simulink model "quadrotor"  (R2016b)
settings: Solver=ode4  StartTime=0.0  StopTime=50  FixedStep=0.01  RelTol=1e-3  EnableMultiTasking=on
values from neighbouring files (symbols this model uses):
  a = 6378137    [Quadparameters.m]
  b = 6356752.3142    [Quadparameters.m]
  d = 7.5*10^(-7)    (= 7.5e-07)    [Quadparameters.m]
  g = 9.81    [Quadparameters.m]
  Ix = 7.5*10^(-3)    (= 0.0075)    [Quadparameters.m]
  Iy = 7.5*10^(-3)    (= 0.0075)    [Quadparameters.m]
  Iz = 1.3*10^(-2)    (= 0.013)    [Quadparameters.m]
  Jr = 6.5*10^(-5)    (= 6.5e-05)    [Quadparameters.m]
  kdp = 0.4    [Quadparameters.m]
  kdps = 0.4    [Quadparameters.m]
  kdt = 0.4    [Quadparameters.m]
  kdz = 20    [Quadparameters.m]
  kpp = 0.8    [Quadparameters.m]
  kpps = 1    [Quadparameters.m]
  kpt = 1.2    [Quadparameters.m]
  kpz = 100    [Quadparameters.m]
  l = 0.23    [Quadparameters.m]
  m = 0.65    [Quadparameters.m]
  NEDDownECEF = [-cos(StartLat)*cos(StartLong) -cos(StartLat)*sin(StartLong) -sin(StartLat)*cos(StartLong)]    [Quadparameters.m]
  NEDEastECEF = [-sin(StartLong) cos(StartLong) 0]    [Quadparameters.m]
  NEDNorthECEF = [-sin(StartLat) 0 cos(StartLat)]    [Quadparameters.m]
  StartECEFX = (a/(sqrt(cos(StartLat)*cos(StartLat)+(b^2/a^2)*sin(StartLat)*sin(StartLat)))+ StartAlt)*cos(StartLat)*cos(StartLong)    [Quadparameters.m]
  StartECEFY = (a/(sqrt(cos(StartLat)*cos(StartLat)+(b^2/a^2)*sin(StartLat)*sin(StartLat)))+ StartAlt)*cos(StartLat)*sin(StartLong)    [Quadparameters.m]
  StartECEFZ = (b/(sqrt((a^2/b^2)*cos(StartLat)*cos(StartLat)+sin(StartLat)*sin(StartLat)))+ StartAlt)*sin(StartLat)    [Quadparameters.m]
undefined symbols (not defined in the file or in its folder): AirSpeed, Altitude, Heading, Latitude, Longitude, Pitch, Roll, VertSpeed
settings Model: ParamWorkspaceSource=ReferencedWorkspace  TunableVars=Ep,Eps,Et,Ez,Gains,Ix,Iy,Iz,Jr,Kdp,Kdps,Kdt,Kdz,Kpp,Kpps,Kpt,Kpz,PhidF,Phiinit,PsidF,Psiinit,ThetadF,Thetainit,Ufour,Uone,Uthree,Utwo,ZdF,Zinit,b,d,g,kdp,kdps,kdt,kdz,kpp,kpps,kpt,kpz,l,m,phitime,psitime,thetatime,tout,yout,ztime  TunableVarsStorageClass=Auto,Auto,Auto,Auto,Auto,Auto,Auto,Auto,Auto,Auto,Auto,Auto,Auto,Auto,Auto,Auto,Auto,Auto,Auto,Auto,Auto,Auto,Auto,Auto,Auto,Auto,Auto,Auto,Auto,Auto,Auto,Auto,Auto,Auto,Auto,Auto,Auto,Auto,Auto,Auto,Auto,Auto,Auto,Auto,Auto,Auto,Auto,Auto  TunableVarsTypeQualifier=,,,,,,,,,,,,,,,,,,,,,,,,,,,,,,,,,,,,,,,,,,,,,,,  Creator=dura_um  LastModifiedBy=leim_ni
settings DataIOCC: LimitDataPoints=on  SaveFormat=Array  SignalLoggingSaveFormat=ModelDataLogs  SaveOutput=off  SignalLogging=off  SaveTime=off
settings OptimizationCC: DefaultParameterBehavior=Inlined  ExpressionDepthLimit=2147483647  InitFltsAndDblsToZero=on  LifeSpan=inf
settings DebuggingCC: UnderspecifiedInitializationDetection=Classic  MergeDetectMultiDrivingBlocksExec=none  SolverPrmCheckMsg=warning  FcnCallInpInsideContextMsg=warning  StateNameClashWarn=warning  StrictBusMsg=Warning  SFUnexpectedBacktrackingDiag=warning  SFNoUnconditionalDefaultTransitionDiag=warning  SFExecutionAtInitializationDiag=none
settings HardwareCC: ProdBitPerPointer=32  ProdBitPerSizeT=32  ProdBitPerPtrDiffT=32  ProdLargestAtomicFloat=None  ProdIntDivRoundTo=Undefined  ProdEndianess=Unspecified  ProdWordSize=32  ProdHWDeviceType=32-bit Generic
settings ModelReferenceCC: PropagateSignalLabelsOutOfModel=off
settings RTWCC: SystemTargetFile=grt_2Simulate.tlc  GenerateMakefile=off  TemplateMakefile=grt_2Simulate_msvc.tmf  Description=2Simulate Target  TargetLang=C++
settings STFCustomTargetCC: ModelReferenceCompliant=off  GeneratePreprocessorConditionals=Disable all  CPPClassGenCompliant=on  SystemTargetFile=grt_2Simulate.tlc
settings GRTTargetCC: TargetLangStandard=C89/C90 (ANSI)  ModelReferenceCompliant=off  ParMdlRefBuildCompliant=off  CompOptLevelCompliant=off  ConcurrentExecutionCompliant=off  GeneratePreprocessorConditionals=Disable all  CombineOutputUpdateFcns=off  MatFileLogging=off  GRTInterface=on  UseToolchainInfoCompliant=off  ExtModeMexFile=noextcomm
settings ConfigComp: CovMetricSettings=dw  CovHtmlReporting=on  CovSaveCumulativeToWorkspaceVar=on  CovSaveSingleToWorkspaceVar=on  CovExternalEMLEnable=off

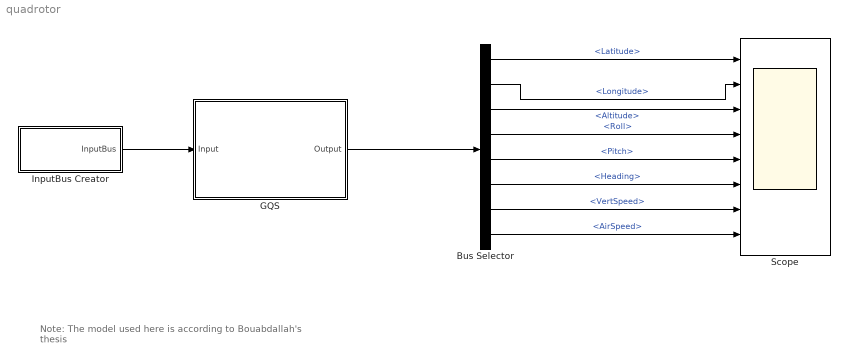
== system quadrotor ==
  note: Note:
      | The model used here is according to Bouabdallah's thesis
  Bus Selector : BusSelector  OutputSignals=Latitude,Longitude,Altitude,Roll,Pitch,Heading,VertSpeed,AirSpeed
  GQS : Subsystem
  "InputBus Creator " : Subsystem
  Scope : Scope  NumInputPorts=8
  wires:
  "InputBus Creator "/1(InputBus) -> GQS/1(Input)
  GQS/1(Output) -> Bus Selector/1
  Bus Selector/3 -> Scope/3  "<Altitude>"
  Bus Selector/4 -> Scope/4  "<Roll>"
  Bus Selector/5 -> Scope/5  "<Pitch>"
  Bus Selector/6 -> Scope/6  "<Heading>"
  Bus Selector/1 -> Scope/1  "<Latitude>"
  Bus Selector/2 -> Scope/2  "<Longitude>"
  Bus Selector/7 -> Scope/7  "<VertSpeed>"
  Bus Selector/8 -> Scope/8  "<AirSpeed>"

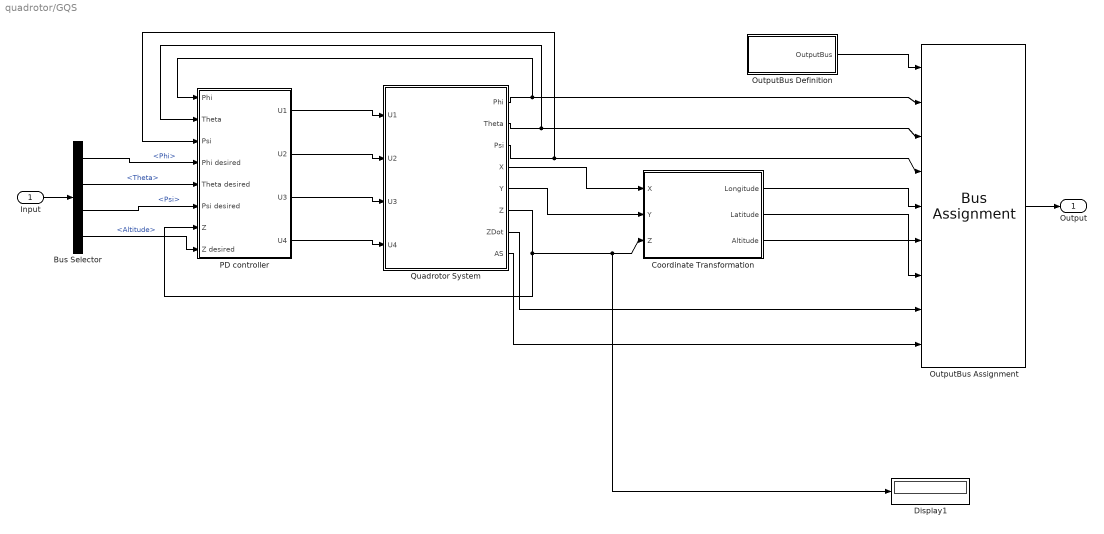
== system quadrotor/GQS ==
  Input : Inport  OutDataTypeStr=Bus: InputVector
  Bus Selector : BusSelector  OutputSignals=Phi,Theta,Psi,Altitude
  Coordinate Transformation : Subsystem
  Display1 : Display
  OutputBus Assignment : BusAssignment  AssignedSignals=Roll,Pitch,Heading,Longitude,Latitude,Altitude,VertSpeed,AirSpeed
  OutputBus Definition : Subsystem
  PD controller : Subsystem
  Quadrotor System : Subsystem
  Output : Outport  OutDataTypeStr=Bus: OutputVector
  wires:
  Quadrotor System/1(Phi) -> PD controller/1(Phi), OutputBus Assignment/2
  Quadrotor System/2(Theta) -> PD controller/2(Theta), OutputBus Assignment/3
  Quadrotor System/6(Z) -> PD controller/7(Z), Display1/1, Coordinate Transformation/3(Z)
  Quadrotor System/3(Psi) -> PD controller/3(Psi), OutputBus Assignment/4
  Bus Selector/4 -> PD controller/8(Z desired)  "<Altitude>"
  PD controller/1(U1) -> Quadrotor System/1(U1)
  OutputBus Assignment/1 -> Output/1
  Bus Selector/1 -> PD controller/4(Phi desired)  "<Phi>"
  Quadrotor System/4(X) -> Coordinate Transformation/1(X)
  OutputBus Definition/1(OutputBus) -> OutputBus Assignment/1
  Quadrotor System/5(Y) -> Coordinate Transformation/2(Y)
  Input/1 -> Bus Selector/1
  Coordinate Transformation/1(Longitude) -> OutputBus Assignment/5
  Coordinate Transformation/3(Altitude) -> OutputBus Assignment/7
  Coordinate Transformation/2(Latitude) -> OutputBus Assignment/6
  PD controller/2(U2) -> Quadrotor System/2(U2)
  PD controller/4(U4) -> Quadrotor System/4(U4)
  Bus Selector/2 -> PD controller/5(Theta desired)  "<Theta>"
  PD controller/3(U3) -> Quadrotor System/3(U3)
  Bus Selector/3 -> PD controller/6(Psi desired)  "<Psi>"
  Quadrotor System/7(ZDot) -> OutputBus Assignment/8
  Quadrotor System/8(AS) -> OutputBus Assignment/9

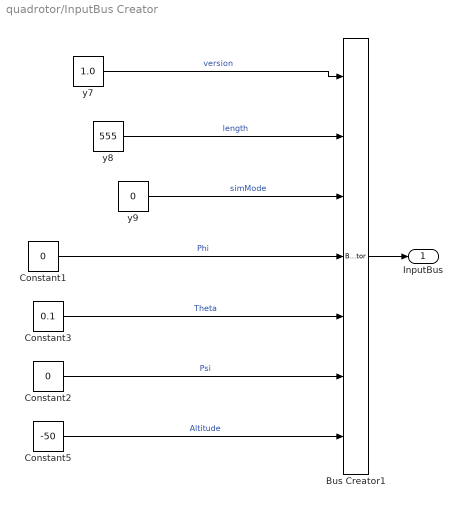
== system quadrotor/InputBus Creator  ==
  Bus Creator1 : BusCreator  Inputs='version','length','simMode','Phi','Theta','Psi','Altitude'  OutDataTypeStr=Bus: InputVector
  Constant1 : Constant  Value=0
  Constant2 : Constant  Value=0
  Constant3 : Constant  Value=0.1
  Constant5 : Constant  Value=-50
  y7 : Constant  Value=1.0  OutDataTypeStr=double
  y8 : Constant  Value=555  OutDataTypeStr=double
  y9 : Constant  Value=0  OutDataTypeStr=double
  InputBus : Outport  OutDataTypeStr=Bus: InputVector
  wires:
  Constant1/1 -> Bus Creator1/4  "Phi"
  Constant3/1 -> Bus Creator1/5  "Theta"
  Constant2/1 -> Bus Creator1/6  "Psi"
  Constant5/1 -> Bus Creator1/7  "Altitude"
  Bus Creator1/1 -> InputBus/1
  y9/1 -> Bus Creator1/3  "simMode"
  y8/1 -> Bus Creator1/2  "length"
  y7/1 -> Bus Creator1/1  "version"

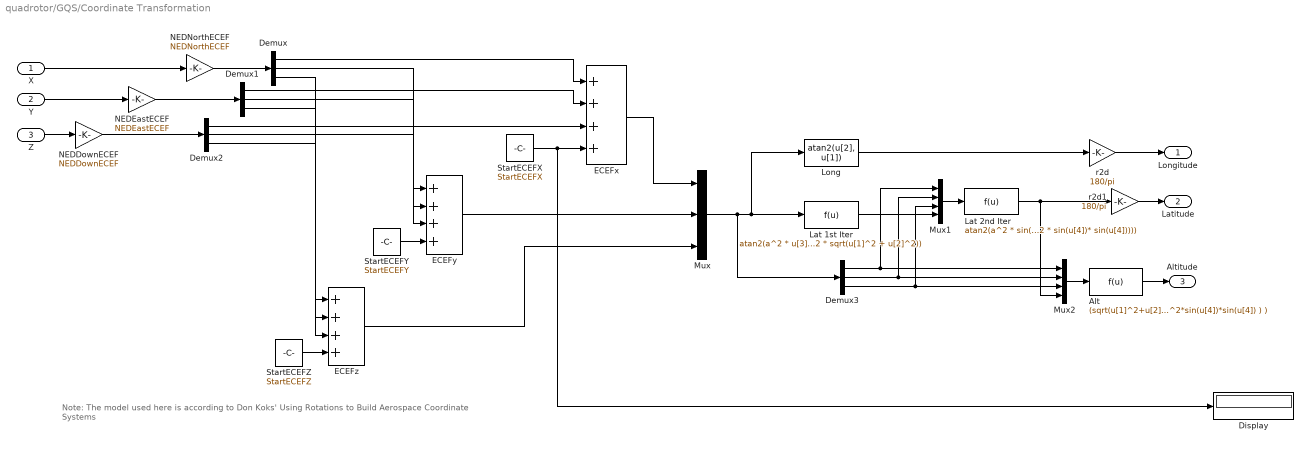
== system quadrotor/GQS/Coordinate Transformation ==
  note: Note:
      | The model used here is according to Don Koks' Using Rotations to Build Aerospace Coordinate Systems
  X : Inport
  Y : Inport  Port=2
  Z : Inport  Port=3
  Alt : Fcn  Expr=(sqrt(u[1]^2+u[2]^2)/cos(u[4]))-( a^2 / sqrt( a^2 * cos(u[4])*cos(u[4])+b^2*sin(u[4])*sin(u[4]) ) )
  Demux{,1..3} (4 alike) : Demux  Outputs=3
  Display : Display
  ECEFx : Sum  Inputs=++++
  ECEFy : Sum  Inputs=++++
  ECEFz : Sum  Inputs=++++
  Lat 1st Iter : Fcn  Expr=atan2(a^2 * u[3], b^2 * sqrt(u[1]^2 + u[2]^2))
  Lat 2nd Iter : Fcn  Expr=atan2(a^2 * sin(u[4])* sin(u[4]),(b^2*sin(u[4])*cos(u[4])+(sqrt(u[1]^2+u[2]^2)*sin(u[4])-u[3]*cos(u[4]))*sqrt(a^2 * cos(u[4])* cos(u[4])+b^2 * sin(u[4])* sin(u[4]))))
  Long : Fcn  Expr=atan2(u[2], u[1])
  Mux : Mux  Inputs=3
  Mux1 : Mux
  Mux2 : Mux
  NEDDownECEF : Gain  Gain=NEDDownECEF
  NEDEastECEF : Gain  Gain=NEDEastECEF
  NEDNorthECEF : Gain  Gain=NEDNorthECEF
  "StartECEFX " : Constant  Value=StartECEFX
  StartECEFY : Constant  Value=StartECEFY
  StartECEFZ : Constant  Value=StartECEFZ
  r2d : Gain  Gain=180/pi
  r2d1 : Gain  Gain=180/pi
  Longitude : Outport
  Latitude : Outport  Port=2
  Altitude : Outport  Port=3
  wires:
  NEDDownECEF/1 -> Demux2/1
  NEDEastECEF/1 -> Demux1/1
  NEDNorthECEF/1 -> Demux/1
  Demux/1 -> ECEFx/1
  Demux/2 -> ECEFy/1
  Demux/3 -> ECEFz/1
  Demux1/1 -> ECEFx/2
  Demux1/2 -> ECEFy/3
  Demux1/3 -> ECEFz/2
  Demux2/1 -> ECEFx/3
  Demux2/2 -> ECEFy/2
  Demux2/3 -> ECEFz/3
  "StartECEFX "/1 -> Display/1, ECEFx/4
  StartECEFY/1 -> ECEFy/4
  StartECEFZ/1 -> ECEFz/4
  ECEFx/1 -> Mux/1
  ECEFy/1 -> Mux/2
  ECEFz/1 -> Mux/3
  Mux/1 -> Lat 1st Iter/1, Long/1, Demux3/1
  Mux1/1 -> Lat 2nd Iter/1
  Lat 2nd Iter/1 -> Mux2/4, r2d1/1
  Mux2/1 -> Alt/1
  Demux3/1 -> Mux2/1, Mux1/1
  Demux3/2 -> Mux2/2, Mux1/2
  Demux3/3 -> Mux2/3, Mux1/3
  Lat 1st Iter/1 -> Mux1/4
  Alt/1 -> Altitude/1
  Long/1 -> r2d/1
  Z/1 -> NEDDownECEF/1
  X/1 -> NEDNorthECEF/1
  Y/1 -> NEDEastECEF/1
  r2d/1 -> Longitude/1
  r2d1/1 -> Latitude/1

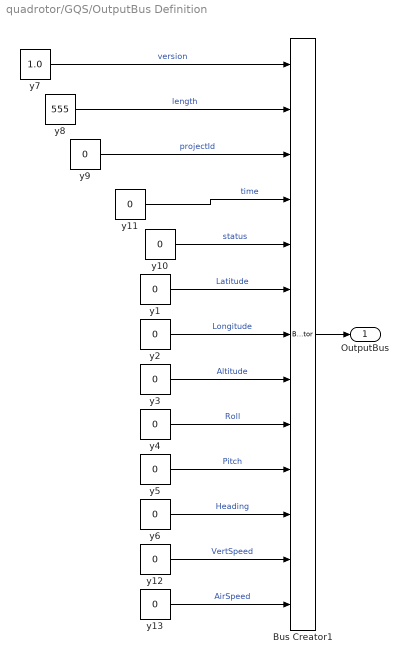
== system quadrotor/GQS/OutputBus Definition ==
  Bus Creator1 : BusCreator  Inputs='version','length','projectId','time','status','Latitude','Longitude','Altitude','Roll','Pitch','Heading','VertSpeed','AirSpeed'  OutDataTypeStr=Bus: OutputVector
  y{1..6,9..13} (11 alike) : Constant  Value=0  OutDataTypeStr=double
  y7 : Constant  Value=1.0  OutDataTypeStr=double
  y8 : Constant  Value=555  OutDataTypeStr=double
  OutputBus : Outport  OutDataTypeStr=Bus: OutputVector
  wires:
  y7/1 -> Bus Creator1/1  "version"
  y8/1 -> Bus Creator1/2  "length"
  y9/1 -> Bus Creator1/3  "projectId"
  Bus Creator1/1 -> OutputBus/1
  y1/1 -> Bus Creator1/6  "Latitude"
  y2/1 -> Bus Creator1/7  "Longitude"
  y3/1 -> Bus Creator1/8  "Altitude"
  y4/1 -> Bus Creator1/9  "Roll"
  y5/1 -> Bus Creator1/10  "Pitch"
  y6/1 -> Bus Creator1/11  "Heading"
  y10/1 -> Bus Creator1/5  "status"
  y11/1 -> Bus Creator1/4  "time"
  y12/1 -> Bus Creator1/12  "VertSpeed"
  y13/1 -> Bus Creator1/13  "AirSpeed"

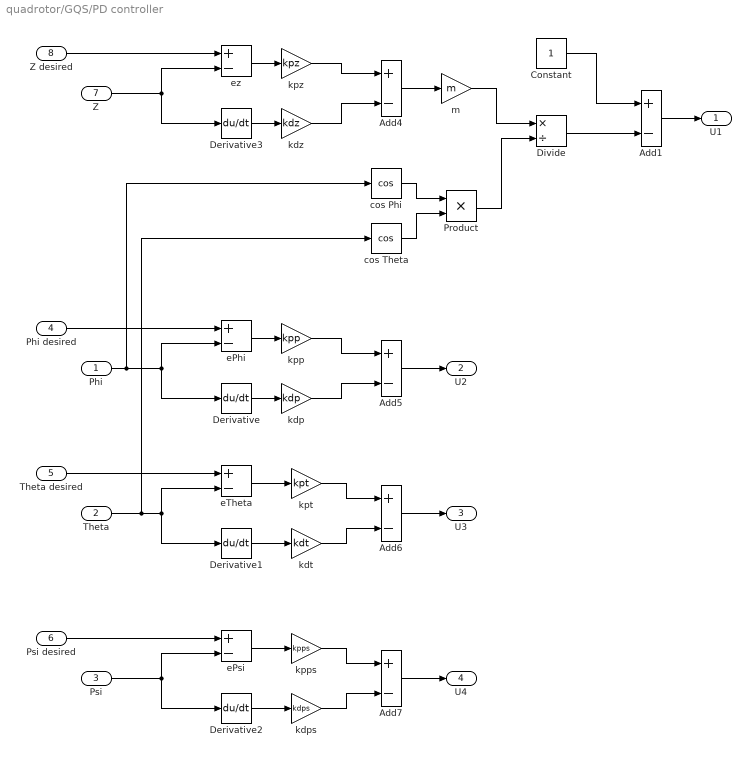
== system quadrotor/GQS/PD controller ==
  Phi : Inport
  Theta : Inport  Port=2
  Psi : Inport  Port=3
  Phi desired : Inport  Port=4
  Theta desired : Inport  Port=5
  Psi desired : Inport  Port=6
  Z : Inport  Port=7
  Z desired : Inport  Port=8
  Add{1,4..7} (5 alike) : Sum  Inputs=+-
  Constant : Constant
  Derivative{,1..3} (4 alike) : Derivative
  Divide : Product  Inputs=*/
  Product : Product  RndMeth=Zero
  cos Phi : Trigonometry  Operator=cos
  cos Theta : Trigonometry  Operator=cos
  ePhi : Sum  Inputs=+-
  ePsi : Sum  Inputs=+-
  eTheta : Sum  Inputs=+-
  ez : Sum  Inputs=+-
  kdp : Gain  Gain=kdp
  kdps : Gain  Gain=kdps
  kdt : Gain  Gain=kdt
  kdz : Gain  Gain=kdz
  kpp : Gain  Gain=kpp
  kpps : Gain  Gain=kpps
  kpt : Gain  Gain=kpt
  kpz : Gain  Gain=kpz
  m : Gain  Gain=m
  U1 : Outport
  U2 : Outport  Port=2
  U3 : Outport  Port=3
  U4 : Outport  Port=4
  wires:
  Phi/1 -> Derivative/1, ePhi/2, cos Phi/1
  Theta/1 -> Derivative1/1, eTheta/2, cos Theta/1
  Psi/1 -> Derivative2/1, ePsi/2
  Phi desired/1 -> ePhi/1
  Theta desired/1 -> eTheta/1
  Psi desired/1 -> ePsi/1
  ePhi/1 -> kpp/1
  Derivative/1 -> kdp/1
  eTheta/1 -> kpt/1
  Derivative1/1 -> kdt/1
  ePsi/1 -> kpps/1
  Derivative2/1 -> kdps/1
  Z/1 -> Derivative3/1, ez/2
  Z desired/1 -> ez/1
  ez/1 -> kpz/1
  Derivative3/1 -> kdz/1
  kpz/1 -> Add4/1
  kdz/1 -> Add4/2
  kpp/1 -> Add5/1
  kdp/1 -> Add5/2
  Add5/1 -> U2/1
  kpt/1 -> Add6/1
  kdt/1 -> Add6/2
  Add6/1 -> U3/1
  kpps/1 -> Add7/1
  kdps/1 -> Add7/2
  Add7/1 -> U4/1
  cos Phi/1 -> Product/1
  cos Theta/1 -> Product/2
  Add4/1 -> m/1
  m/1 -> Divide/1
  Product/1 -> Divide/2
  Constant/1 -> Add1/1
  Divide/1 -> Add1/2
  Add1/1 -> U1/1

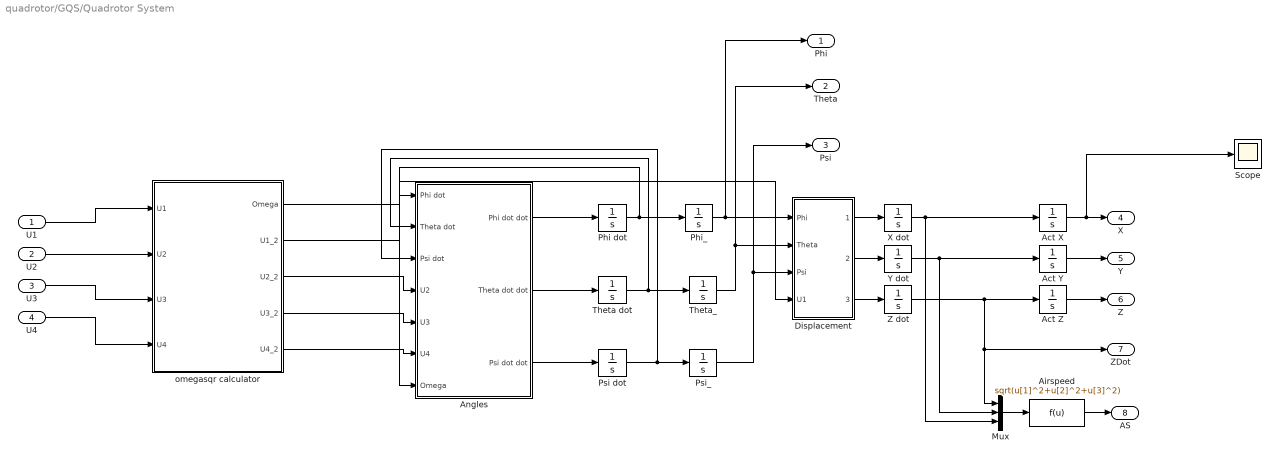
== system quadrotor/GQS/Quadrotor System ==
  U1 : Inport
  U2 : Inport  Port=2
  U3 : Inport  Port=3
  U4 : Inport  Port=4
  Act X : Integrator
  Act Y : Integrator
  Act Z : Integrator
  Airspeed : Fcn  Expr=sqrt(u[1]^2+u[2]^2+u[3]^2)
  Angles : Subsystem
  Displacement : Subsystem
  Mux : Mux  Inputs=3
  Phi dot : Integrator
  "Phi_ " : Integrator  ZeroCross=off
  Psi dot : Integrator  ZeroCross=off
  Psi_ : Integrator  ZeroCross=off
  Scope : Scope
  Theta dot : Integrator  ZeroCross=off
  Theta_ : Integrator  ZeroCross=off
  X dot : Integrator
  Y dot : Integrator
  Z dot : Integrator
  omegasqr calculator : Subsystem
  Phi : Outport
  Theta : Outport  Port=2
  Psi : Outport  Port=3
  X : Outport  Port=4
  Y : Outport  Port=5
  Z : Outport  Port=6
  ZDot : Outport  Port=7
  AS : Outport  Port=8
  wires:
  Angles/1(Phi dot dot) -> Phi dot/1
  Angles/2(Theta dot dot) -> Theta dot/1
  Angles/3(Psi dot dot) -> Psi dot/1
  Phi dot/1 -> Angles/1(Phi dot), "Phi_ "/1
  Theta dot/1 -> Angles/2(Theta dot), Theta_/1
  Psi dot/1 -> Angles/3(Psi dot), Psi_/1
  "Phi_ "/1 -> Displacement/1(Phi), Phi/1
  Theta_/1 -> Displacement/2(Theta), Theta/1
  Psi_/1 -> Displacement/3(Psi), Psi/1
  Displacement/1(x dotdot) -> X dot/1
  X dot/1 -> Act X/1, Mux/3
  Y dot/1 -> Act Y/1, Mux/2
  Displacement/2(y dotdot) -> Y dot/1
  Z dot/1 -> Act Z/1, ZDot/1, Mux/1
  Displacement/3(z dotdot) -> Z dot/1
  Act X/1 -> Scope/1, X/1
  Act Y/1 -> Y/1
  Act Z/1 -> Z/1
  U1/1 -> omegasqr calculator/1(U1)
  U2/1 -> omegasqr calculator/2(U2)
  U3/1 -> omegasqr calculator/3(U3)
  U4/1 -> omegasqr calculator/4(U4)
  omegasqr calculator/2(U1_2) -> Displacement/4(U1)
  omegasqr calculator/1(Omega) -> Angles/7(Omega)
  omegasqr calculator/3(U2_2) -> Angles/4(U2)
  omegasqr calculator/4(U3_2) -> Angles/5(U3)
  omegasqr calculator/5(U4_2) -> Angles/6(U4)
  Mux/1 -> Airspeed/1
  Airspeed/1 -> AS/1

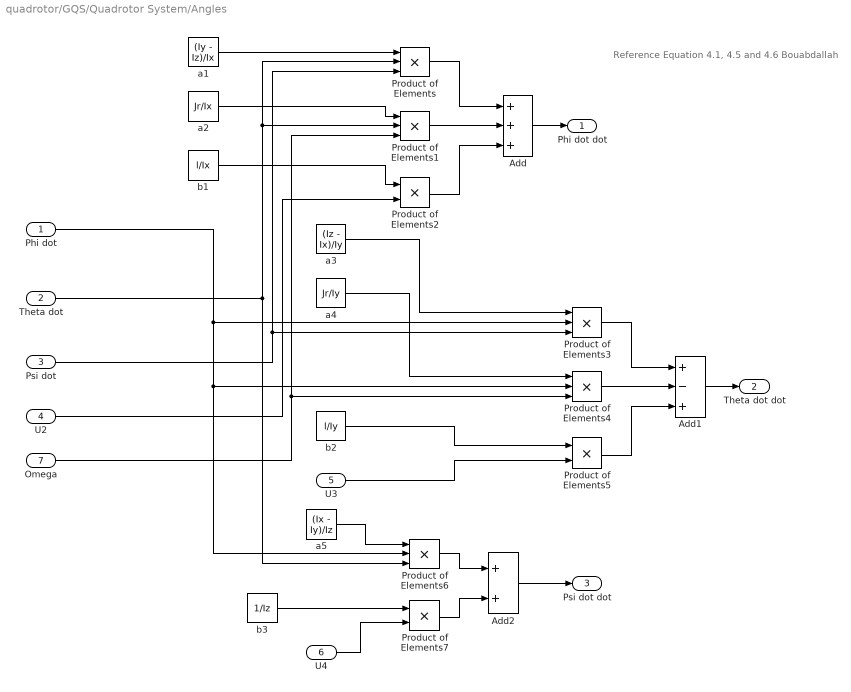
== system quadrotor/GQS/Quadrotor System/Angles ==
  note: Reference Equation 4.1, 4.5 and 4.6 Bouabdallah
  Phi dot : Inport
  Theta dot : Inport  Port=2
  Psi dot : Inport  Port=3
  U2 : Inport  Port=4
  U3 : Inport  Port=5
  U4 : Inport  Port=6
  Omega : Inport  Port=7
  Add : Sum  Inputs=+++
  Add1 : Sum  Inputs=+-+
  Add2 : Sum
  Product of Elements{,1,3..4,6} (5 alike) : Product  Inputs=3
  Product of Elements2 : Product
  Product of Elements5 : Product
  Product of Elements7 : Product
  a1 : Constant  Value=(Iy - Iz)/Ix
  a2 : Constant  Value=Jr/Ix
  a3 : Constant  Value=(Iz - Ix)/Iy
  a4 : Constant  Value=Jr/Iy
  a5 : Constant  Value=(Ix - Iy)/Iz
  b1 : Constant  Value=l/Ix
  b2 : Constant  Value=l/Iy
  b3 : Constant  Value=1/Iz
  Phi dot dot : Outport
  Theta dot dot : Outport  Port=2
  Psi dot dot : Outport  Port=3
  wires:
  Product of Elements/1 -> Add/1
  Product of Elements1/1 -> Add/2
  Product of Elements2/1 -> Add/3
  Add/1 -> Phi dot dot/1
  a1/1 -> Product of Elements/1
  Theta dot/1 -> Product of Elements/2, Product of Elements1/2, Product of Elements6/3
  Psi dot/1 -> Product of Elements/3, Product of Elements3/3
  a2/1 -> Product of Elements1/1
  b1/1 -> Product of Elements2/1
  U2/1 -> Product of Elements2/2
  Omega/1 -> Product of Elements1/3, Product of Elements4/3
  Product of Elements3/1 -> Add1/1
  Product of Elements4/1 -> Add1/2
  Product of Elements5/1 -> Add1/3
  Add1/1 -> Theta dot dot/1
  a3/1 -> Product of Elements3/1
  a4/1 -> Product of Elements4/1
  b2/1 -> Product of Elements5/1
  U3/1 -> Product of Elements5/2
  Phi dot/1 -> Product of Elements3/2, Product of Elements4/2, Product of Elements6/2
  Product of Elements6/1 -> Add2/1
  Product of Elements7/1 -> Add2/2
  Add2/1 -> Psi dot dot/1
  U4/1 -> Product of Elements7/2
  b3/1 -> Product of Elements7/1
  a5/1 -> Product of Elements6/1

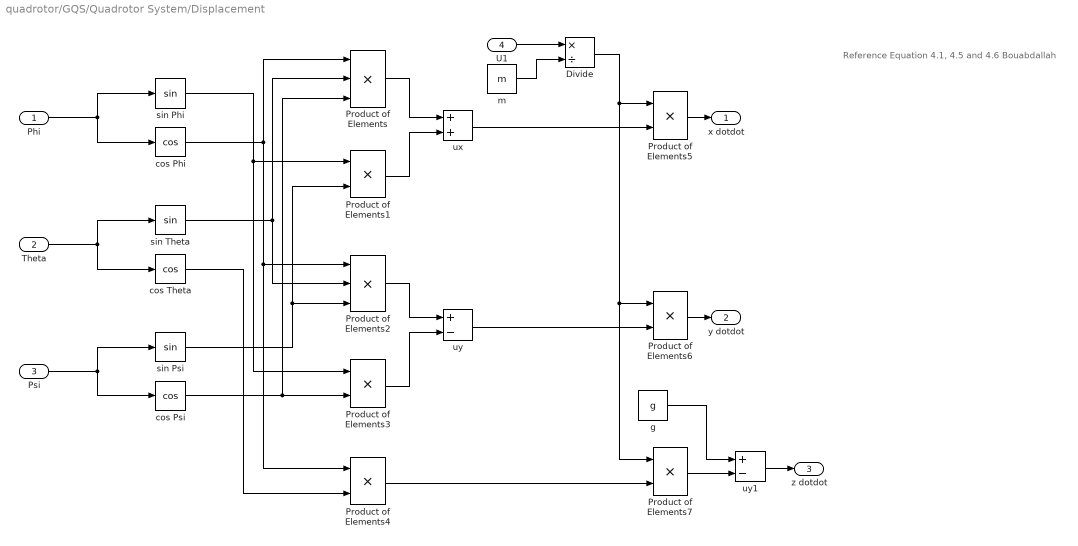
== system quadrotor/GQS/Quadrotor System/Displacement ==
  note: Reference Equation 4.1, 4.5 and 4.6 Bouabdallah
  Phi : Inport
  Theta : Inport  Port=2
  Psi : Inport  Port=3
  U1 : Inport  Port=4
  Divide : Product  Inputs=*/
  Product of Elements : Product  Inputs=3
  Product of Elements{1,3..7} (6 alike) : Product
  Product of Elements2 : Product  Inputs=3
  cos Phi : Trigonometry  Operator=cos
  cos Psi : Trigonometry  Operator=cos
  cos Theta : Trigonometry  Operator=cos
  g : Constant  Value=g
  m : Constant  Value=m
  sin Phi : Trigonometry
  sin Psi : Trigonometry
  sin Theta : Trigonometry
  ux : Sum
  uy : Sum  Inputs=+-
  uy1 : Sum  Inputs=+-
  x dotdot : Outport
  y dotdot : Outport  Port=2
  z dotdot : Outport  Port=3
  wires:
  Phi/1 -> sin Phi/1, cos Phi/1
  Theta/1 -> sin Theta/1, cos Theta/1
  Psi/1 -> sin Psi/1, cos Psi/1
  sin Theta/1 -> Product of Elements/2, Product of Elements2/2
  cos Psi/1 -> Product of Elements/3, Product of Elements3/2
  cos Phi/1 -> Product of Elements/1, Product of Elements2/1, Product of Elements4/1
  sin Phi/1 -> Product of Elements1/1, Product of Elements3/1
  sin Psi/1 -> Product of Elements1/2, Product of Elements2/3
  Product of Elements/1 -> ux/1
  Product of Elements1/1 -> ux/2
  ux/1 -> Product of Elements5/2
  Product of Elements2/1 -> uy/1
  Product of Elements3/1 -> uy/2
  uy/1 -> Product of Elements6/2
  cos Theta/1 -> Product of Elements4/2
  Product of Elements4/1 -> Product of Elements7/2
  U1/1 -> Divide/1
  m/1 -> Divide/2
  Divide/1 -> Product of Elements5/1, Product of Elements6/1, Product of Elements7/1
  Product of Elements5/1 -> x dotdot/1
  Product of Elements6/1 -> y dotdot/1
  uy1/1 -> z dotdot/1
  Product of Elements7/1 -> uy1/2
  g/1 -> uy1/1

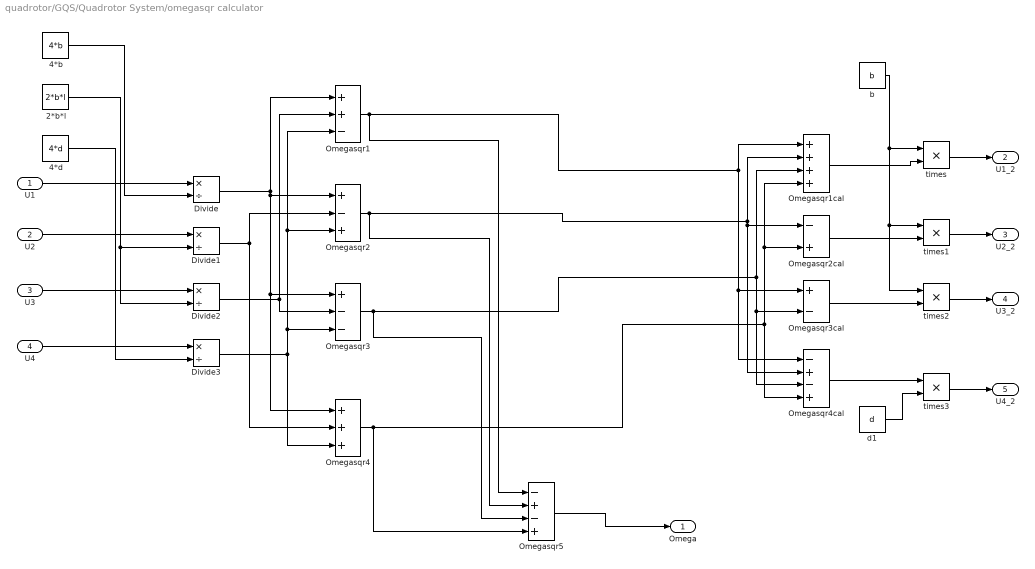
== system quadrotor/GQS/Quadrotor System/omegasqr calculator ==
  U1 : Inport
  U2 : Inport  Port=2
  U3 : Inport  Port=3
  U4 : Inport  Port=4
  2*b*l : Constant  Value=2*b*l
  4*b : Constant  Value=4*b
  4*d : Constant  Value=4*d
  Divide{,1..3} (4 alike) : Product  Inputs=*/
  Omegasqr1 : Sum  Inputs=++-
  Omegasqr1cal : Sum  Inputs=++++
  Omegasqr2 : Sum  Inputs=+-+
  Omegasqr2cal : Sum  Inputs=-+
  Omegasqr3 : Sum  Inputs=+--
  Omegasqr3cal : Sum  Inputs=+-
  Omegasqr4 : Sum  Inputs=+++
  Omegasqr4cal : Sum  Inputs=-+-+
  Omegasqr5 : Sum  Inputs=-+-+
  b : Constant  Value=b
  d1 : Constant  Value=d
  times{,1..3} (4 alike) : Product  Inputs=**
  Omega : Outport
  U1_2 : Outport  Port=2
  U2_2 : Outport  Port=3
  U3_2 : Outport  Port=4
  U4_2 : Outport  Port=5
  wires:
  U1/1 -> Divide/1
  4*b/1 -> Divide/2
  U2/1 -> Divide1/1
  2*b*l/1 -> Divide1/2, Divide2/2
  U3/1 -> Divide2/1
  U4/1 -> Divide3/1
  4*d/1 -> Divide3/2
  Divide/1 -> Omegasqr1/1, Omegasqr2/1, Omegasqr3/1, Omegasqr4/1
  Divide2/1 -> Omegasqr1/2, Omegasqr3/2
  Divide3/1 -> Omegasqr1/3, Omegasqr2/3, Omegasqr3/3, Omegasqr4/3
  Divide1/1 -> Omegasqr2/2, Omegasqr4/2
  Omegasqr1/1 -> Omegasqr5/1, Omegasqr1cal/1, Omegasqr3cal/1, Omegasqr4cal/1
  Omegasqr2/1 -> Omegasqr5/2, Omegasqr1cal/2, Omegasqr2cal/1, Omegasqr4cal/2
  Omegasqr3/1 -> Omegasqr5/3, Omegasqr1cal/3, Omegasqr3cal/2, Omegasqr4cal/3
  Omegasqr4/1 -> Omegasqr5/4, Omegasqr1cal/4, Omegasqr2cal/2, Omegasqr4cal/4
  b/1 -> times/1, times1/1, times2/1
  Omegasqr1cal/1 -> times/2
  Omegasqr2cal/1 -> times1/2
  Omegasqr3cal/1 -> times2/2
  Omegasqr4cal/1 -> times3/1
  d1/1 -> times3/2
  times/1 -> U1_2/1
  times1/1 -> U2_2/1
  times3/1 -> U4_2/1
  times2/1 -> U3_2/1
  Omegasqr5/1 -> Omega/1
